simulink model "sampleModel7293_pp_1_1"  (R2018a)
settings: Solver=VariableStepAuto  StartTime=0.0  StopTime=10.0  RelTol=1e-3
undefined symbols (not defined in the file): DiscIntNeverNeededParam
libraries: simulink x367
(part 4 of 12)

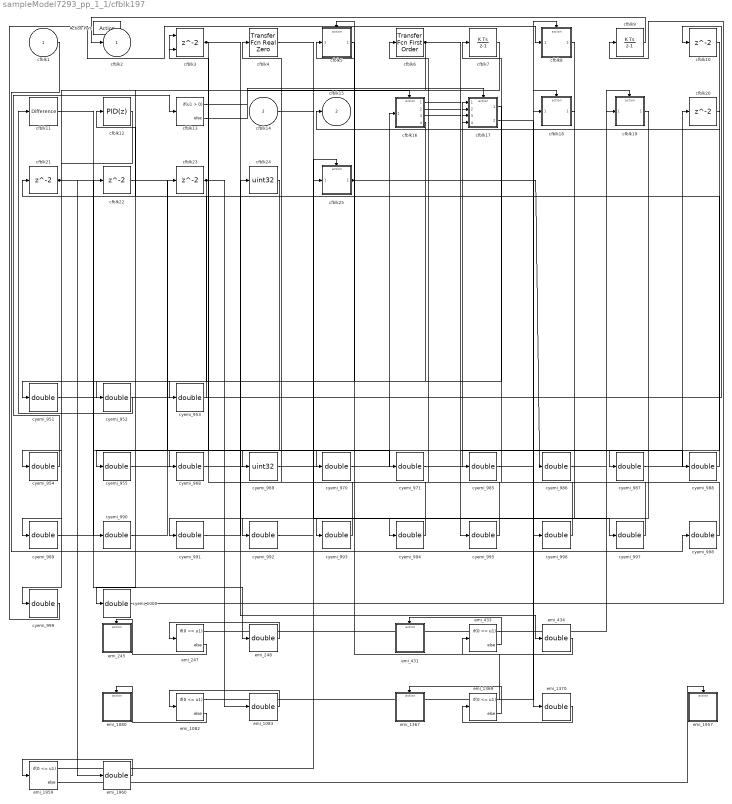
== system sampleModel7293_pp_1_1/cfblk197 ==
  cfblk1 : Inport
  cfblk14 : Inport  Port=2
  Action Port : ActionPort  ActionType=else
  cfblk{10,20..23} (5 alike) : Delay
  cfblk11 : simulink/Discrete/Difference  ICPrevInput=0.0  OutMin=[]  OutMax=[]  OutDataTypeStr=double  OutputDataTypeScalingMode=double  OutDataType=fixdt(1, 16)  OutScaling=2^-10  DoSatur=off
  cfblk12 : simulink/Continuous/PID Controller  Controller=PID  TimeDomain=Discrete-time  SampleTime=-1  IntegratorMethod=Forward Euler  FilterMethod=Forward Euler  Form=Parallel  UseFilter=on  ControllerParametersSource=internal  P=1  I=1  D=0  N=100  InitialConditionSource=internal  InitialConditionForIntegrator=0  InitialConditionForFilter=0  ExternalReset=none  LimitOutput=off  UpperSaturationLimit=inf  LowerSaturationLimit=-inf  LinearizeAsGain=off  AntiWindupMode=none  Kb=1  TrackingMode=off  Kt=1  PParamMin=[]  PParamMax=[]  IParamMin=[]  IParamMax=[]  DParamMin=[]  DParamMax=[]  NParamMin=[]  NParamMax=[]  KbParamMin=[]  KbParamMax=[]  KtParamMin=[]  KtParamMax=[]  POutMin=[]  POutMax=[]  IOutMin=[]  IOutMax=[]  DOutMin=[]  DOutMax=[]  NOutMin=[]  NOutMax=[]  KbOutMin=[]  KbOutMax=[]  KtOutMin=[]  KtOutMax=[]  IntegratorOutMin=[]  IntegratorOutMax=[]  FilterOutMin=[]  FilterOutMax=[]  SumOutMin=[]  SumOutMax=[]  SumI1OutMin=[]  SumI1OutMax=[]  SumI2OutMin=[]  SumI2OutMax=[]  SumI3OutMin=[]  SumI3OutMax=[]  SumDOutMin=[]  SumDOutMax=[]  SaturationOutMin=[]  SaturationOutMax=[]  IntegratorContinuousStateAttributes=''  IntegratorStateMustResolveToSignalObject=off  IntegratorRTWStateStorageClass=Auto  FilterContinuousStateAttributes=''  FilterStateMustResolveToSignalObject=off  FilterRTWStateStorageClass=Auto  DifferentiatorICPrevScaledInput=0  DifferentiatorOutMin=[]  DifferentiatorOutMax=[]  FilterDiffOutCoefMin=[]  FilterDiffOutCoefMax=[]  SumDenOutMin=[]  SumDenOutMax=[]  SumNumOutMin=[]  SumNumOutMax=[]  ReciprocalOutMin=[]  ReciprocalOutMax=[]  DivideOutMin=[]  DivideOutMax=[]  TunerSelectOption=Transfer Function Based (PID Tuner App)
  cfblk13 : If  SampleTime=1
  cfblk16 : Subsystem  TreatAsAtomicUnit=on
  cfblk17 : Subsystem  TreatAsAtomicUnit=on
  cfblk18 : Subsystem  TreatAsAtomicUnit=on
  cfblk19 : Subsystem  TreatAsAtomicUnit=on
  cfblk24 : DataTypeConversion  OutDataTypeStr=uint32
  cfblk25 : Subsystem  TreatAsAtomicUnit=on
  cfblk3 : Delay  ShowEnablePort=on
      settings: InputPortMap=u0,e6
  cfblk4 : simulink/Discrete/Transfer Fcn Real Zero  ZeroZ=0.75  ICPrevInput=0.0  DoSatur=off
      settings: SourceProductName=Simulink  SourceProductBaseCode=SL
  cfblk5 : Subsystem  TreatAsAtomicUnit=on
  cfblk6 : simulink/Discrete/Transfer Fcn First Order  PoleZ=0.95  ICPrevOutput=0.0  DoSatur=off
      settings: SourceProductName=Simulink
  cfblk7 : DiscreteIntegrator  SampleTime=-1  OutDataTypeStr=double  ICPrevOutput=DiscIntNeverNeededParam  ICPrevScaledInput=DiscIntNeverNeededParam
  cfblk8 : Subsystem  TreatAsAtomicUnit=on
  cfblk9 : DiscreteIntegrator  SampleTime=-1  OutDataTypeStr=double  ICPrevOutput=DiscIntNeverNeededParam  ICPrevScaledInput=DiscIntNeverNeededParam
  cyemi_{951..955,968,970..971,985..1000} (24 alike) : DataTypeConversion  OutDataTypeStr=double
  cyemi_969 : DataTypeConversion  OutDataTypeStr=uint32
  emi_1080 : Subsystem  TreatAsAtomicUnit=on
  emi_{247,433,1082,1369,1959} (5 alike) : If  IfExpression=0 <= u1
  emi_{248,434,1083,1370,1960} (5 alike) : DataTypeConversion  OutDataTypeStr=double
  emi_1367 : Subsystem  TreatAsAtomicUnit=on
  emi_1957 : Subsystem  TreatAsAtomicUnit=on
  emi_245 : Subsystem  TreatAsAtomicUnit=on
  emi_431 : Subsystem  TreatAsAtomicUnit=on
  cfblk2 : Outport
  cfblk15 : Outport  Port=2
  wires:
  cfblk10/1 -> cfblk15/1
  cfblk9/1 -> cfblk2/1
  cfblk6/1 -> cyemi_987/1, cyemi_999/1
  cfblk13/1 -> cfblk16/Action
  cfblk13/2 -> cfblk17/Action
  cyemi_951/1 -> cfblk10/1
  cfblk17/1(cfblk2) -> cyemi_951/1
  cyemi_952/1 -> cfblk11/1
  cyemi_953/1 -> cfblk12/1
  cfblk16/4(cfblk13) -> cyemi_953/1
  cyemi_954/1 -> cfblk13/1
  cfblk23/1 -> cyemi_954/1, emi_1083/1
  cyemi_955/1 -> cfblk16/1(cfblk1)
  cfblk20/1 -> cyemi_955/1
  cyemi_968/1 -> cfblk17/1(cfblk1)
  cfblk3/1 -> cyemi_968/1, emi_434/1
  cyemi_969/1 -> cfblk17/2(cfblk12)
  cfblk24/1 -> cyemi_969/1
  cyemi_970/1 -> cfblk17/3(cfblk13)
  cfblk22/1 -> cyemi_970/1
  cyemi_971/1 -> cfblk17/4(cfblk14)
  cfblk21/1 -> cyemi_971/1, emi_248/1, emi_1960/1
  cfblk16/1(cfblk2) -> cyemi_985/1
  cyemi_987/1 -> cfblk20/1
  cyemi_988/1 -> cfblk21/1
  cfblk16/3(cfblk12) -> cyemi_988/1
  cyemi_989/1 -> cfblk22/1
  cfblk12/1 -> cyemi_989/1
  cyemi_990/1 -> cfblk23/1
  cfblk11/1 -> cyemi_990/1
  cyemi_991/1 -> cfblk24/1
  cyemi_993/1 -> cfblk3/1
  cyemi_994/1 -> cfblk3/2
  cfblk14/1 -> cyemi_994/1
  cyemi_995/1 -> cfblk4/1
  cfblk16/2(cfblk11) -> cyemi_995/1
  cfblk17/2(cfblk15) -> cyemi_996/1
  cyemi_997/1 -> cfblk6/1
  cfblk4/1 -> cyemi_997/1
  cyemi_998/1 -> cfblk7/1
  cfblk1/1 -> cyemi_998/1
  cyemi_1000/1 -> cfblk9/1
  cfblk7/1 -> cyemi_1000/1
  cyemi_999/1 -> cfblk8/1(emi_243)
  cfblk8/1(emi_244) -> cyemi_992/1
  emi_247/1 -> cfblk8/Action
  emi_247/2 -> emi_245/Action
  emi_248/1 -> emi_247/1
  cyemi_986/1 -> cfblk19/1(emi_429)
  cfblk19/1(emi_430) -> cyemi_991/1
  emi_433/1 -> cfblk19/Action
  emi_433/2 -> emi_431/Action
  emi_434/1 -> emi_433/1
  cyemi_985/1 -> cfblk18/1(emi_1078)
  cfblk18/1(emi_1079) -> cyemi_993/1
  emi_1082/1 -> cfblk18/Action
  emi_1082/2 -> emi_1080/Action
  emi_1083/1 -> emi_1082/1
  cyemi_996/1 -> cfblk5/1(emi_1365)
  cfblk5/1(emi_1366) -> cyemi_952/1
  emi_1369/1 -> cfblk5/Action
  emi_1369/2 -> emi_1367/Action
  emi_1370/1 -> emi_1369/1
  cyemi_992/1 -> cfblk25/1(emi_1955)
  cfblk25/1(emi_1956) -> emi_1370/1, cyemi_986/1
  emi_1959/1 -> cfblk25/Action
  emi_1959/2 -> emi_1957/Action
  emi_1960/1 -> emi_1959/1

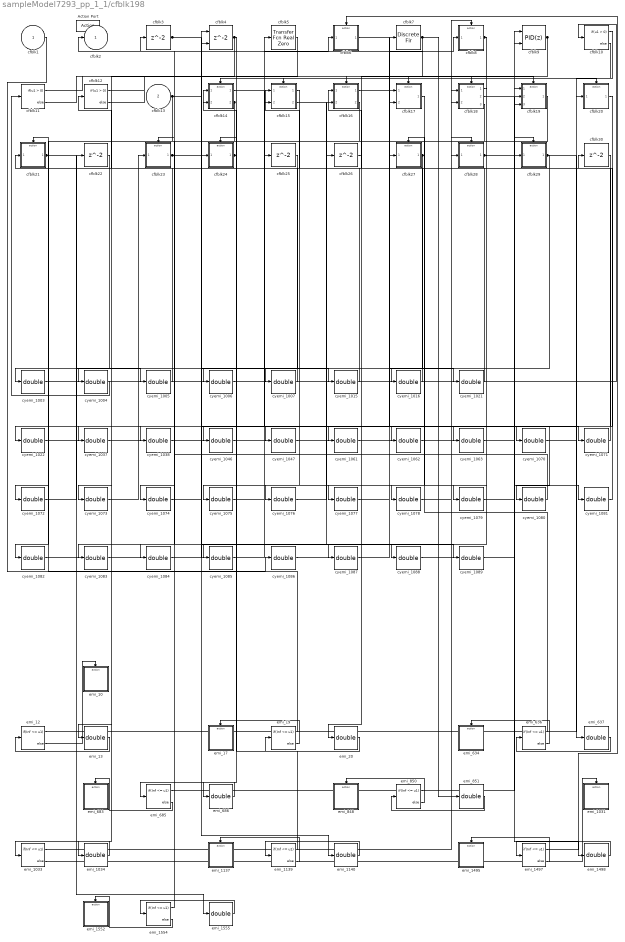
== system sampleModel7293_pp_1_1/cfblk198 ==
  cfblk1 : Inport
  cfblk13 : Inport  Port=2
  Action Port : ActionPort  ActionType=then
  cfblk10 : If  SampleTime=1
  cfblk11 : If  SampleTime=1
  cfblk12 : If  SampleTime=1
  cfblk14 : Subsystem  TreatAsAtomicUnit=on
  cfblk15 : Subsystem  TreatAsAtomicUnit=on
  cfblk16 : Subsystem  TreatAsAtomicUnit=on
  cfblk17 : Subsystem  TreatAsAtomicUnit=on
  cfblk18 : Subsystem  TreatAsAtomicUnit=on
  cfblk19 : Subsystem  TreatAsAtomicUnit=on
  cfblk20 : Subsystem  TreatAsAtomicUnit=on
  cfblk21 : Subsystem  TreatAsAtomicUnit=on
  cfblk{3,22,25..26,30} (5 alike) : Delay
  cfblk23 : Subsystem  TreatAsAtomicUnit=on
  cfblk24 : Subsystem  TreatAsAtomicUnit=on
  cfblk27 : Subsystem  TreatAsAtomicUnit=on
  cfblk28 : Subsystem  TreatAsAtomicUnit=on
  cfblk29 : Subsystem  TreatAsAtomicUnit=on
  cfblk4 : Delay  ShowEnablePort=on
      settings: InputPortMap=u0,e6
  cfblk5 : simulink/Discrete/Transfer Fcn Real Zero  ZeroZ=0.75  ICPrevInput=0.0  DoSatur=off
      settings: SourceProductName=Simulink  SourceProductBaseCode=SL
  cfblk6 : Subsystem  TreatAsAtomicUnit=on
  cfblk7 : DiscreteFir
  cfblk8 : Subsystem  TreatAsAtomicUnit=on
  cfblk9 : simulink/Continuous/PID Controller (2DOF)  Controller=PID  TimeDomain=Discrete-time  SampleTime=-1  IntegratorMethod=Forward Euler  FilterMethod=Forward Euler  Form=Parallel  UseFilter=on  ControllerParametersSource=internal  P=1  I=1  D=0  N=100  b=1  c=1  InitialConditionSource=internal  InitialConditionForIntegrator=0  InitialConditionForFilter=0  ExternalReset=none  LimitOutput=off  UpperSaturationLimit=inf  LowerSaturationLimit=-inf  LinearizeAsGain=off  AntiWindupMode=none  Kb=1  TrackingMode=off  Kt=1  PParamMin=[]  PParamMax=[]  IParamMin=[]  IParamMax=[]  DParamMin=[]  DParamMax=[]  NParamMin=[]  NParamMax=[]  bParamMin=[]  bParamMax=[]  cParamMin=[]  cParamMax=[]  KbParamMin=[]  KbParamMax=[]  KtParamMin=[]  KtParamMax=[]  POutMin=[]  POutMax=[]  IOutMin=[]  IOutMax=[]  DOutMin=[]  DOutMax=[]  NOutMin=[]  NOutMax=[]  bOutMin=[]  bOutMax=[]  cOutMin=[]  cOutMax=[]  KbOutMin=[]  KbOutMax=[]  KtOutMin=[]  KtOutMax=[]  IntegratorOutMin=[]  IntegratorOutMax=[]  FilterOutMin=[]  FilterOutMax=[]  SumOutMin=[]  SumOutMax=[]  Sum1OutMin=[]  Sum1OutMax=[]  Sum2OutMin=[]  Sum2OutMax=[]  Sum3OutMin=[]  Sum3OutMax=[]  SumI1OutMin=[]  SumI1OutMax=[]  SumI2OutMin=[]  SumI2OutMax=[]  SumI3OutMin=[]  SumI3OutMax=[]  SumDOutMin=[]  SumDOutMax=[]  SaturationOutMin=[]  SaturationOutMax=[]  IntegratorContinuousStateAttributes=''  IntegratorStateMustResolveToSignalObject=off  IntegratorRTWStateStorageClass=Auto  FilterContinuousStateAttributes=''  FilterStateMustResolveToSignalObject=off  FilterRTWStateStorageClass=Auto  DifferentiatorICPrevScaledInput=0  DifferentiatorOutMin=[]  DifferentiatorOutMax=[]  FilterDiffOutCoefMin=[]  FilterDiffOutCoefMax=[]  SumDenOutMin=[]  SumDenOutMax=[]  SumNumOutMin=[]  SumNumOutMax=[]  ReciprocalOutMin=[]  ReciprocalOutMax=[]  DivideOutMin=[]  DivideOutMax=[]  TunerSelectOption=Transfer Function Based (PID Tuner App)
  cyemi_{1003..1007,1015..1016,1021..1022,1037..1038,1046..1047,1061..1063,1070..1089} (36 alike) : DataTypeConversion  OutDataTypeStr=double
  emi_10 : Subsystem  TreatAsAtomicUnit=on
  emi_1031 : Subsystem  TreatAsAtomicUnit=on
  emi_{12,19,636,685,850,1033,1139,1497,1554} (9 alike) : If  IfExpression=Inf <= u1
  emi_{13,20,637,686,851,1034,1140,1498,1555} (9 alike) : DataTypeConversion  OutDataTypeStr=double
  emi_1137 : Subsystem  TreatAsAtomicUnit=on
  emi_1495 : Subsystem  TreatAsAtomicUnit=on
  emi_1552 : Subsystem  TreatAsAtomicUnit=on
  emi_17 : Subsystem  TreatAsAtomicUnit=on
  emi_634 : Subsystem  TreatAsAtomicUnit=on
  emi_683 : Subsystem  TreatAsAtomicUnit=on
  emi_848 : Subsystem  TreatAsAtomicUnit=on
  cfblk2 : Outport
  wires:
  cfblk7/1 -> cfblk2/1, emi_20/1, emi_851/1
  cfblk3/1 -> cyemi_1047/1, cyemi_1063/1
  cfblk9/1 -> cyemi_1079/1, cyemi_1087/1
  cfblk13/1 -> cyemi_1004/1, cyemi_1015/1, cyemi_1089/1
  cfblk14/2(cfblk11) -> cyemi_1073/1, cyemi_1074/1
  cfblk10/1 -> cfblk14/Action
  cfblk10/2 -> cfblk15/Action
  cfblk11/1 -> cfblk16/Action
  cfblk11/2 -> cfblk17/Action
  cfblk12/1 -> cfblk18/Action
  cfblk12/2 -> cfblk19/Action
  cyemi_1003/1 -> cfblk10/1
  cyemi_1004/1 -> cfblk11/1
  cyemi_1005/1 -> cfblk12/1
  cyemi_1006/1 -> cfblk14/1(cfblk1)
  cfblk5/1 -> cyemi_1006/1
  cyemi_1007/1 -> cfblk14/2(cfblk10)
  cfblk25/1 -> cyemi_1007/1
  cyemi_1015/1 -> cfblk15/1(cfblk1)
  cyemi_1016/1 -> cfblk15/2(cfblk6)
  cyemi_1021/1 -> cfblk16/1(cfblk1)
  cyemi_1022/1 -> cfblk16/2(cfblk14)
  cyemi_1037/1 -> cfblk17/1(cfblk1)
  cfblk18/3(cfblk16) -> cyemi_1037/1
  cyemi_1038/1 -> cfblk17/2(cfblk10)
  cyemi_1046/1 -> cfblk18/1(cfblk1)
  cyemi_1047/1 -> cfblk18/2(cfblk14)
  cyemi_1061/1 -> cfblk19/1(cfblk1)
  cfblk26/1 -> cyemi_1061/1
  cyemi_1062/1 -> cfblk19/2(cfblk9)
  cyemi_1063/1 -> cfblk19/3(cfblk10)
  cfblk16/1(cfblk2) -> cyemi_1070/1
  cfblk14/1(cfblk2) -> cyemi_1071/1
  cyemi_1072/1 -> cfblk22/1
  cfblk19/1(cfblk2) -> cyemi_1072/1
  cyemi_1075/1 -> cfblk25/1
  cfblk15/1(cfblk2) -> cyemi_1075/1
  cyemi_1076/1 -> cfblk26/1
  cfblk17/1(cfblk2) -> cyemi_1078/1
  cyemi_1080/1 -> cfblk3/1
  cfblk30/1 -> cyemi_1080/1
  cyemi_1081/1 -> cfblk30/1
  cfblk18/2(cfblk15) -> cyemi_1081/1
  cyemi_1082/1 -> cfblk4/1
  cfblk22/1 -> cyemi_1082/1
  cyemi_1083/1 -> cfblk4/2
  cfblk18/1(cfblk2) -> cyemi_1083/1
  cyemi_1084/1 -> cfblk5/1
  cfblk16/2(cfblk15) -> cyemi_1084/1
  cfblk4/1 -> cyemi_1085/1, emi_13/1
  cyemi_1086/1 -> cfblk7/1
  cfblk1/1 -> cyemi_1086/1
  cyemi_1088/1 -> cfblk9/1
  cfblk15/2(cfblk7) -> cyemi_1088/1
  cyemi_1089/1 -> cfblk9/2
  cyemi_1070/1 -> cfblk20/1(emi_8)
  cfblk20/1(emi_9) -> cyemi_1046/1
  emi_12/1 -> cfblk20/Action
  emi_12/2 -> emi_10/Action
  emi_13/1 -> emi_12/1
  cyemi_1071/1 -> cfblk21/1(emi_15)
  cfblk21/1(emi_16) -> cyemi_1005/1, emi_1555/1
  emi_19/1 -> cfblk21/Action
  emi_19/2 -> emi_17/Action
  emi_20/1 -> emi_19/1
  cyemi_1077/1 -> cfblk27/1(emi_632)
  cfblk27/1(emi_633) -> cyemi_1038/1, emi_1034/1
  emi_636/1 -> cfblk27/Action
  emi_636/2 -> emi_634/Action
  emi_637/1 -> emi_636/1
  cyemi_1079/1 -> cfblk29/1(emi_681)
  cfblk29/1(emi_682) -> emi_637/1, cyemi_1016/1
  emi_685/1 -> cfblk29/Action
  emi_685/2 -> emi_683/Action
  emi_686/1 -> emi_685/1
  cyemi_1087/1 -> cfblk8/1(emi_846)
  cfblk8/1(emi_847) -> cyemi_1077/1, cyemi_1076/1
  emi_850/1 -> cfblk8/Action
  emi_850/2 -> emi_848/Action
  emi_851/1 -> emi_850/1
  cyemi_1078/1 -> cfblk28/1(emi_1029)
  cfblk28/1(emi_1030) -> cyemi_1062/1, emi_1498/1
  emi_1033/1 -> cfblk28/Action
  emi_1033/2 -> emi_1031/Action
  emi_1034/1 -> emi_1033/1
  cyemi_1074/1 -> cfblk24/1(emi_1135)
  cfblk24/1(emi_1136) -> emi_686/1, cyemi_1003/1
  emi_1139/1 -> cfblk24/Action
  emi_1139/2 -> emi_1137/Action
  emi_1140/1 -> emi_1139/1
  cyemi_1085/1 -> cfblk6/1(emi_1493)
  cfblk6/1(emi_1494) -> cyemi_1021/1
  emi_1497/1 -> cfblk6/Action
  emi_1497/2 -> emi_1495/Action
  emi_1498/1 -> emi_1497/1
  cyemi_1073/1 -> cfblk23/1(emi_1550)
  cfblk23/1(emi_1551) -> emi_1140/1, cyemi_1022/1
  emi_1554/1 -> cfblk23/Action
  emi_1554/2 -> emi_1552/Action
  emi_1555/1 -> emi_1554/1

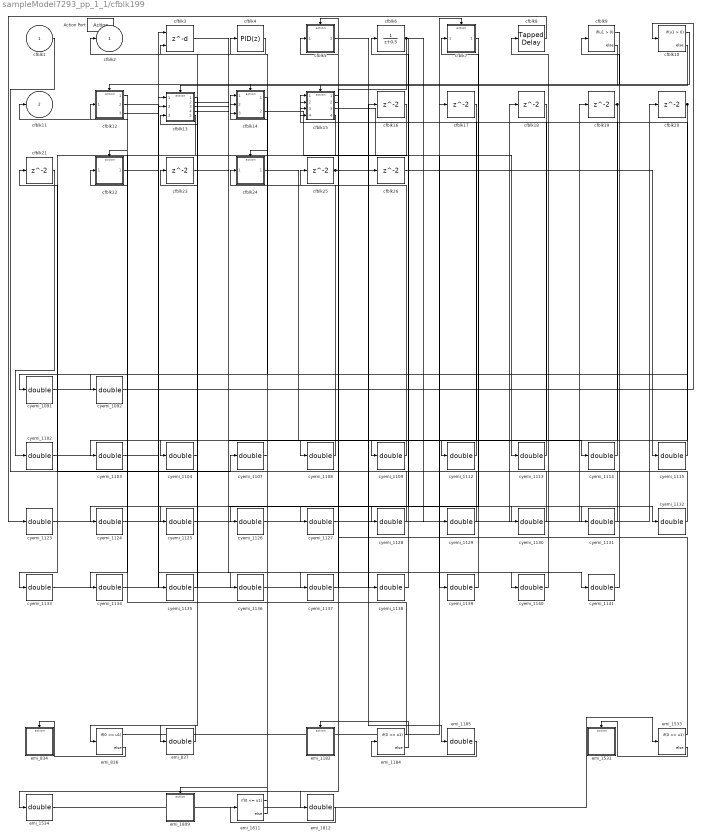
== system sampleModel7293_pp_1_1/cfblk199 ==
  cfblk1 : Inport
  Action Port : ActionPort  ActionType=else
  cfblk10 : If  SampleTime=1
  cfblk12 : Subsystem  TreatAsAtomicUnit=on
  cfblk13 : Subsystem  TreatAsAtomicUnit=on
  cfblk14 : Subsystem  TreatAsAtomicUnit=on
  cfblk15 : Subsystem  TreatAsAtomicUnit=on
  cfblk{16..21,23,25..26} (9 alike) : Delay
  cfblk22 : Subsystem  TreatAsAtomicUnit=on
  cfblk24 : Subsystem  TreatAsAtomicUnit=on
  cfblk3 : Delay  DelayLengthSource=Input port
      settings: InputPortMap=u0,p1
  cfblk4 : simulink/Continuous/PID Controller  Controller=PID  TimeDomain=Discrete-time  SampleTime=-1  IntegratorMethod=Forward Euler  FilterMethod=Forward Euler  Form=Parallel  UseFilter=on  ControllerParametersSource=internal  P=1  I=1  D=0  N=100  InitialConditionSource=internal  InitialConditionForIntegrator=0  InitialConditionForFilter=0  ExternalReset=none  LimitOutput=off  UpperSaturationLimit=inf  LowerSaturationLimit=-inf  LinearizeAsGain=off  AntiWindupMode=none  Kb=1  TrackingMode=off  Kt=1  PParamMin=[]  PParamMax=[]  IParamMin=[]  IParamMax=[]  DParamMin=[]  DParamMax=[]  NParamMin=[]  NParamMax=[]  KbParamMin=[]  KbParamMax=[]  KtParamMin=[]  KtParamMax=[]  POutMin=[]  POutMax=[]  IOutMin=[]  IOutMax=[]  DOutMin=[]  DOutMax=[]  NOutMin=[]  NOutMax=[]  KbOutMin=[]  KbOutMax=[]  KtOutMin=[]  KtOutMax=[]  IntegratorOutMin=[]  IntegratorOutMax=[]  FilterOutMin=[]  FilterOutMax=[]  SumOutMin=[]  SumOutMax=[]  SumI1OutMin=[]  SumI1OutMax=[]  SumI2OutMin=[]  SumI2OutMax=[]  SumI3OutMin=[]  SumI3OutMax=[]  SumDOutMin=[]  SumDOutMax=[]  SaturationOutMin=[]  SaturationOutMax=[]  IntegratorContinuousStateAttributes=''  IntegratorStateMustResolveToSignalObject=off  IntegratorRTWStateStorageClass=Auto  FilterContinuousStateAttributes=''  FilterStateMustResolveToSignalObject=off  FilterRTWStateStorageClass=Auto  DifferentiatorICPrevScaledInput=0  DifferentiatorOutMin=[]  DifferentiatorOutMax=[]  FilterDiffOutCoefMin=[]  FilterDiffOutCoefMax=[]  SumDenOutMin=[]  SumDenOutMax=[]  SumNumOutMin=[]  SumNumOutMax=[]  ReciprocalOutMin=[]  ReciprocalOutMax=[]  DivideOutMin=[]  DivideOutMax=[]  TunerSelectOption=Transfer Function Based (PID Tuner App)
  cfblk5 : Subsystem  TreatAsAtomicUnit=on
  cfblk6 : DiscreteTransferFcn
  cfblk7 : Subsystem  TreatAsAtomicUnit=on
  cfblk8 : simulink/Discrete/Tapped Delay  vinit=0.0  samptime=-1  NumDelays=1  DelayOrder=Oldest  includeCurrent=off
  cfblk9 : If  SampleTime=1
  cyemi_{1091..1092,1102..1104,1107..1109,1112..1115,1123..1141} (31 alike) : DataTypeConversion  OutDataTypeStr=double
  emi_1182 : Subsystem  TreatAsAtomicUnit=on
  emi_{836,1184,1533,1811} (4 alike) : If  IfExpression=0 <= u1
  emi_{837,1185,1534,1812} (4 alike) : DataTypeConversion  OutDataTypeStr=double
  emi_1531 : Subsystem  TreatAsAtomicUnit=on
  emi_1809 : Subsystem  TreatAsAtomicUnit=on
  emi_834 : Subsystem  TreatAsAtomicUnit=on
  cfblk2 : Outport
  cfblk11 : Outport  Port=2
  wires:
  cfblk12/1(cfblk2) -> cfblk11/1
  cfblk6/1 -> cyemi_1128/1, cyemi_1129/1, emi_1534/1
  cfblk4/1 -> cfblk2/1
  cfblk9/1 -> cfblk12/Action
  cfblk9/2 -> cfblk13/Action
  cfblk10/1 -> cfblk14/Action
  cfblk10/2 -> cfblk15/Action
  cyemi_1091/1 -> cfblk10/1
  cfblk20/1 -> cyemi_1091/1, emi_837/1
  cyemi_1092/1 -> cfblk12/1(cfblk1)
  cfblk14/1(cfblk2) -> cyemi_1092/1
  cyemi_1102/1 -> cfblk13/1(cfblk1)
  cfblk21/1 -> cyemi_1102/1
  cyemi_1103/1 -> cfblk13/2(cfblk5)
  cfblk18/1 -> cyemi_1103/1
  cyemi_1104/1 -> cfblk13/3(cfblk6)
  cfblk16/1 -> cyemi_1104/1
  cyemi_1107/1 -> cfblk14/1(cfblk1)
  cfblk1/1 -> cyemi_1107/1
  cyemi_1108/1 -> cfblk14/2(cfblk5)
  cfblk23/1 -> cyemi_1108/1
  cyemi_1109/1 -> cfblk14/3(cfblk6)
  cfblk19/1 -> cyemi_1109/1, emi_1812/1
  cyemi_1112/1 -> cfblk15/1(cfblk1)
  cfblk17/1 -> cyemi_1112/1
  cyemi_1113/1 -> cfblk15/2(cfblk9)
  cfblk14/2(cfblk7) -> cyemi_1113/1
  cyemi_1114/1 -> cfblk15/3(cfblk10)
  cyemi_1115/1 -> cfblk15/4(cfblk11)
  cfblk26/1 -> cyemi_1115/1
  cyemi_1123/1 -> cfblk16/1
  cfblk8/1 -> cyemi_1123/1
  cyemi_1124/1 -> cfblk17/1
  cfblk13/1(cfblk2) -> cyemi_1124/1
  cyemi_1125/1 -> cfblk18/1
  cfblk15/1(cfblk2) -> cyemi_1125/1
  cyemi_1126/1 -> cfblk19/1
  cfblk15/2(cfblk12) -> cyemi_1126/1
  cyemi_1127/1 -> cfblk20/1
  cyemi_1128/1 -> cfblk21/1
  cyemi_1130/1 -> cfblk23/1
  cfblk13/2(cfblk7) -> cyemi_1130/1
  cfblk13/3(cfblk8) -> cyemi_1131/1
  cyemi_1132/1 -> cfblk25/1
  cfblk13/4(cfblk9) -> cyemi_1132/1
  cyemi_1133/1 -> cfblk26/1
  cfblk13/5(cfblk10) -> cyemi_1133/1
  cyemi_1134/1 -> cfblk3/1
  cfblk15/4(cfblk14) -> cyemi_1134/1
  cyemi_1135/1 -> cfblk3/2
  cyemi_1136/1 -> cfblk4/1
  cfblk12/2(cfblk9) -> cyemi_1136/1
  cfblk3/1 -> cyemi_1137/1
  cyemi_1138/1 -> cfblk6/1
  cfblk15/3(cfblk13) -> cyemi_1139/1
  cyemi_1140/1 -> cfblk8/1
  cfblk12/3(cfblk10) -> cyemi_1140/1
  cyemi_1141/1 -> cfblk9/1
  cfblk25/1 -> cyemi_1141/1, emi_1185/1
  cyemi_1139/1 -> cfblk7/1(emi_832)
  cfblk7/1(emi_833) -> cyemi_1127/1
  emi_836/1 -> cfblk7/Action
  emi_836/2 -> emi_834/Action
  emi_837/1 -> emi_836/1
  cyemi_1129/1 -> cfblk22/1(emi_1180)
  cfblk22/1(emi_1181) -> cyemi_1135/1
  emi_1184/1 -> cfblk22/Action
  emi_1184/2 -> emi_1182/Action
  emi_1185/1 -> emi_1184/1
  cyemi_1137/1 -> cfblk5/1(emi_1529)
  cfblk5/1(emi_1530) -> cyemi_1138/1
  emi_1533/1 -> cfblk5/Action
  emi_1533/2 -> emi_1531/Action
  emi_1534/1 -> emi_1533/1
  cyemi_1131/1 -> cfblk24/1(emi_1807)
  cfblk24/1(emi_1808) -> cyemi_1114/1
  emi_1811/1 -> cfblk24/Action
  emi_1811/2 -> emi_1809/Action
  emi_1812/1 -> emi_1811/1

== system sampleModel7293_pp_1_1/cfblk2 ==
  emi_1245 : Inport
  Action Port : ActionPort  ActionType=then
  cfblk2 : DiscreteIntegrator  OutDataTypeStr=double  ICPrevOutput=DiscIntNeverNeededParam  ICPrevScaledInput=DiscIntNeverNeededParam
  emi_1246 : Outport
  wires:
  emi_1245/1 -> cfblk2/1
  cfblk2/1 -> emi_1246/1

== system sampleModel7293_pp_1_1/cfblk200 ==
  cfblk1 : Inport
  Action Port : ActionPort  ActionType=then
  cfblk10 : If  SampleTime=1
  cfblk11 : Subsystem  TreatAsAtomicUnit=on
  cfblk12 : Subsystem  TreatAsAtomicUnit=on
  cfblk13 : Delay
  cfblk14 : Delay
  cfblk3 : Subsystem  TreatAsAtomicUnit=on
  cfblk4 : Subsystem  TreatAsAtomicUnit=on
  cfblk5 : Delay  DelayLengthSource=Input port
      settings: InputPortMap=u0,p1
  cfblk6 : Delay
  cfblk7 : UnitDelay  SampleTime=-1
  cfblk8 : simulink/Continuous/PID Controller (2DOF)  Controller=PID  TimeDomain=Discrete-time  SampleTime=-1  IntegratorMethod=Forward Euler  FilterMethod=Forward Euler  Form=Parallel  UseFilter=on  ControllerParametersSource=internal  P=1  I=1  D=0  N=100  b=1  c=1  InitialConditionSource=internal  InitialConditionForIntegrator=0  InitialConditionForFilter=0  ExternalReset=none  LimitOutput=off  UpperSaturationLimit=inf  LowerSaturationLimit=-inf  LinearizeAsGain=off  AntiWindupMode=none  Kb=1  TrackingMode=off  Kt=1  PParamMin=[]  PParamMax=[]  IParamMin=[]  IParamMax=[]  DParamMin=[]  DParamMax=[]  NParamMin=[]  NParamMax=[]  bParamMin=[]  bParamMax=[]  cParamMin=[]  cParamMax=[]  KbParamMin=[]  KbParamMax=[]  KtParamMin=[]  KtParamMax=[]  POutMin=[]  POutMax=[]  IOutMin=[]  IOutMax=[]  DOutMin=[]  DOutMax=[]  NOutMin=[]  NOutMax=[]  bOutMin=[]  bOutMax=[]  cOutMin=[]  cOutMax=[]  KbOutMin=[]  KbOutMax=[]  KtOutMin=[]  KtOutMax=[]  IntegratorOutMin=[]  IntegratorOutMax=[]  FilterOutMin=[]  FilterOutMax=[]  SumOutMin=[]  SumOutMax=[]  Sum1OutMin=[]  Sum1OutMax=[]  Sum2OutMin=[]  Sum2OutMax=[]  Sum3OutMin=[]  Sum3OutMax=[]  SumI1OutMin=[]  SumI1OutMax=[]  SumI2OutMin=[]  SumI2OutMax=[]  SumI3OutMin=[]  SumI3OutMax=[]  SumDOutMin=[]  SumDOutMax=[]  SaturationOutMin=[]  SaturationOutMax=[]  IntegratorContinuousStateAttributes=''  IntegratorStateMustResolveToSignalObject=off  IntegratorRTWStateStorageClass=Auto  FilterContinuousStateAttributes=''  FilterStateMustResolveToSignalObject=off  FilterRTWStateStorageClass=Auto  DifferentiatorICPrevScaledInput=0  DifferentiatorOutMin=[]  DifferentiatorOutMax=[]  FilterDiffOutCoefMin=[]  FilterDiffOutCoefMax=[]  SumDenOutMin=[]  SumDenOutMax=[]  SumNumOutMin=[]  SumNumOutMax=[]  ReciprocalOutMin=[]  ReciprocalOutMax=[]  DivideOutMin=[]  DivideOutMax=[]  TunerSelectOption=Transfer Function Based (PID Tuner App)
  cfblk9 : UnitDelay  SampleTime=-1
  cyemi_{1145..1146,1157..1158,1169..1179} (15 alike) : DataTypeConversion  OutDataTypeStr=double
  emi_641 : Subsystem  TreatAsAtomicUnit=on
  emi_643 : If  IfExpression=Inf <= u1
  emi_644 : DataTypeConversion  OutDataTypeStr=double
  emi_926 : Subsystem  TreatAsAtomicUnit=on
  emi_928 : If  IfExpression=Inf <= u1
  emi_929 : DataTypeConversion  OutDataTypeStr=double
  cfblk2 : Outport
  wires:
  cfblk9/1 -> cfblk2/1, emi_929/1
  cfblk5/1 -> cyemi_1158/1, cyemi_1176/1
  cfblk6/1 -> cyemi_1174/1, cyemi_1179/1, emi_644/1
  cfblk10/1 -> cfblk11/Action
  cfblk10/2 -> cfblk12/Action
  cyemi_1145/1 -> cfblk10/1
  cyemi_1146/1 -> cfblk11/1(cfblk1)
  cfblk14/1 -> cyemi_1146/1
  cyemi_1157/1 -> cfblk12/1(cfblk1)
  cyemi_1158/1 -> cfblk12/2(cfblk9)
  cyemi_1169/1 -> cfblk13/1
  cfblk8/1 -> cyemi_1169/1
  cyemi_1170/1 -> cfblk14/1
  cfblk7/1 -> cyemi_1171/1
  cfblk11/1(cfblk2) -> cyemi_1172/1
  cyemi_1173/1 -> cfblk5/1
  cfblk13/1 -> cyemi_1173/1
  cyemi_1174/1 -> cfblk5/2
  cyemi_1175/1 -> cfblk6/1
  cfblk1/1 -> cyemi_1175/1
  cyemi_1176/1 -> cfblk7/1
  cyemi_1177/1 -> cfblk8/1
  cfblk12/1(cfblk2) -> cyemi_1177/1
  cyemi_1178/1 -> cfblk8/2
  cyemi_1179/1 -> cfblk9/1
  cyemi_1172/1 -> cfblk4/1(emi_639)
  cfblk4/1(emi_640) -> cyemi_1170/1
  emi_643/1 -> cfblk4/Action
  emi_643/2 -> emi_641/Action
  emi_644/1 -> emi_643/1
  cyemi_1171/1 -> cfblk3/1(emi_924)
  cfblk3/1(emi_925) -> cyemi_1178/1, cyemi_1157/1, cyemi_1145/1
  emi_928/1 -> cfblk3/Action
  emi_928/2 -> emi_926/Action
  emi_929/1 -> emi_928/1

== system sampleModel7293_pp_1_1/cfblk201 ==
  cfblk1 : Inport
  Action Port : ActionPort  ActionType=else
  cfblk10 : simulink/Discrete/Transfer Fcn First Order  PoleZ=0.95  ICPrevOutput=0.0  DoSatur=off
      settings: SourceProductName=Simulink
  cfblk11 : DiscreteIntegrator  SampleTime=-1  OutDataTypeStr=double  ICPrevOutput=DiscIntNeverNeededParam  ICPrevScaledInput=DiscIntNeverNeededParam
  cfblk12 : Subsystem  TreatAsAtomicUnit=on
  cfblk13 : simulink/Discrete/Transfer Fcn Real Zero  ZeroZ=0.75  ICPrevInput=0.0  DoSatur=off
      settings: SourceProductName=Simulink  SourceProductBaseCode=SL
  cfblk14 : DiscreteStateSpace  SampleTime=-1
  cfblk15 : Delay
  cfblk3 : UnitDelay  SampleTime=-1
  cfblk4 : Subsystem  TreatAsAtomicUnit=on
  cfblk5 : DiscreteFir
  cfblk6 : DiscreteTransferFcn
  cfblk7 : Subsystem  TreatAsAtomicUnit=on
  cfblk8 : Subsystem  TreatAsAtomicUnit=on
  cfblk9 : Delay
  cyemi_{1181..1194} (14 alike) : DataTypeConversion  OutDataTypeStr=double
  emi_1261 : Subsystem  TreatAsAtomicUnit=on
  emi_{477,914,1263,1312} (4 alike) : If  IfExpression=0 <= u1
  emi_{478,915,1264,1313} (4 alike) : DataTypeConversion  OutDataTypeStr=double
  emi_1310 : Subsystem  TreatAsAtomicUnit=on
  emi_475 : Subsystem  TreatAsAtomicUnit=on
  emi_912 : Subsystem  TreatAsAtomicUnit=on
  cfblk2 : Outport
  wires:
  cfblk1/1 -> cyemi_1189/1, cyemi_1190/1
  cfblk13/1 -> cfblk2/1
  cyemi_1181/1 -> cfblk10/1
  cfblk14/1 -> cyemi_1181/1
  cyemi_1182/1 -> cfblk11/1
  cfblk6/1 -> cyemi_1183/1
  cyemi_1184/1 -> cfblk13/1
  cyemi_1185/1 -> cfblk14/1
  cyemi_1186/1 -> cfblk15/1
  cfblk9/1 -> cyemi_1186/1, emi_1313/1
  cyemi_1187/1 -> cfblk3/1
  cfblk11/1 -> cyemi_1187/1
  cfblk3/1 -> cyemi_1188/1
  cyemi_1190/1 -> cfblk5/1
  cyemi_1191/1 -> cfblk6/1
  cfblk5/1 -> cyemi_1192/1, emi_915/1
  cfblk15/1 -> cyemi_1193/1, emi_1264/1
  cyemi_1194/1 -> cfblk9/1
  cfblk10/1 -> cyemi_1194/1
  cyemi_1188/1 -> cfblk4/1(emi_472)
  cyemi_1189/1 -> cfblk4/2(emi_473)
  cfblk4/1(emi_474) -> cyemi_1184/1
  emi_477/1 -> cfblk4/Action
  emi_477/2 -> emi_475/Action
  emi_478/1 -> emi_477/1
  cyemi_1192/1 -> cfblk7/1(emi_910)
  cfblk7/1(emi_911) -> cyemi_1191/1
  emi_914/1 -> cfblk7/Action
  emi_914/2 -> emi_912/Action
  emi_915/1 -> emi_914/1
  cyemi_1183/1 -> cfblk12/1(emi_1259)
  cfblk12/1(emi_1260) -> cyemi_1182/1
  emi_1263/1 -> cfblk12/Action
  emi_1263/2 -> emi_1261/Action
  emi_1264/1 -> emi_1263/1
  cyemi_1193/1 -> cfblk8/1(emi_1308)
  cfblk8/1(emi_1309) -> emi_478/1, cyemi_1185/1
  emi_1312/1 -> cfblk8/Action
  emi_1312/2 -> emi_1310/Action
  emi_1313/1 -> emi_1312/1

== system sampleModel7293_pp_1_1/cfblk202 ==
  cfblk1 : Inport
  Action Port : ActionPort  ActionType=then
  cfblk10 : Subsystem  TreatAsAtomicUnit=on
  cfblk11 : DiscreteTransferFcn
  cfblk12 : Delay
  cfblk13 : Subsystem  TreatAsAtomicUnit=on
  cfblk3 : Subsystem  TreatAsAtomicUnit=on
  cfblk4 : Subsystem  TreatAsAtomicUnit=on
  cfblk5 : simulink/Continuous/PID Controller (2DOF)  Controller=PID  TimeDomain=Discrete-time  SampleTime=-1  IntegratorMethod=Forward Euler  FilterMethod=Forward Euler  Form=Parallel  UseFilter=on  ControllerParametersSource=internal  P=1  I=1  D=0  N=100  b=1  c=1  InitialConditionSource=internal  InitialConditionForIntegrator=0  InitialConditionForFilter=0  ExternalReset=none  LimitOutput=off  UpperSaturationLimit=inf  LowerSaturationLimit=-inf  LinearizeAsGain=off  AntiWindupMode=none  Kb=1  TrackingMode=off  Kt=1  PParamMin=[]  PParamMax=[]  IParamMin=[]  IParamMax=[]  DParamMin=[]  DParamMax=[]  NParamMin=[]  NParamMax=[]  bParamMin=[]  bParamMax=[]  cParamMin=[]  cParamMax=[]  KbParamMin=[]  KbParamMax=[]  KtParamMin=[]  KtParamMax=[]  POutMin=[]  POutMax=[]  IOutMin=[]  IOutMax=[]  DOutMin=[]  DOutMax=[]  NOutMin=[]  NOutMax=[]  bOutMin=[]  bOutMax=[]  cOutMin=[]  cOutMax=[]  KbOutMin=[]  KbOutMax=[]  KtOutMin=[]  KtOutMax=[]  IntegratorOutMin=[]  IntegratorOutMax=[]  FilterOutMin=[]  FilterOutMax=[]  SumOutMin=[]  SumOutMax=[]  Sum1OutMin=[]  Sum1OutMax=[]  Sum2OutMin=[]  Sum2OutMax=[]  Sum3OutMin=[]  Sum3OutMax=[]  SumI1OutMin=[]  SumI1OutMax=[]  SumI2OutMin=[]  SumI2OutMax=[]  SumI3OutMin=[]  SumI3OutMax=[]  SumDOutMin=[]  SumDOutMax=[]  SaturationOutMin=[]  SaturationOutMax=[]  IntegratorContinuousStateAttributes=''  IntegratorStateMustResolveToSignalObject=off  IntegratorRTWStateStorageClass=Auto  FilterContinuousStateAttributes=''  FilterStateMustResolveToSignalObject=off  FilterRTWStateStorageClass=Auto  DifferentiatorICPrevScaledInput=0  DifferentiatorOutMin=[]  DifferentiatorOutMax=[]  FilterDiffOutCoefMin=[]  FilterDiffOutCoefMax=[]  SumDenOutMin=[]  SumDenOutMax=[]  SumNumOutMin=[]  SumNumOutMax=[]  ReciprocalOutMin=[]  ReciprocalOutMax=[]  DivideOutMin=[]  DivideOutMax=[]  TunerSelectOption=Transfer Function Based (PID Tuner App)
  cfblk6 : UnitDelay  SampleTime=-1
  cfblk7 : Subsystem  TreatAsAtomicUnit=on
  cfblk8 : Delay  DelayLengthSource=Input port
      settings: InputPortMap=u0,p1
  cfblk9 : simulink/Continuous/PID Controller (2DOF)  Controller=PID  TimeDomain=Discrete-time  SampleTime=-1  IntegratorMethod=Forward Euler  FilterMethod=Forward Euler  Form=Parallel  UseFilter=on  ControllerParametersSource=internal  P=1  I=1  D=0  N=100  b=1  c=1  InitialConditionSource=internal  InitialConditionForIntegrator=0  InitialConditionForFilter=0  ExternalReset=none  LimitOutput=off  UpperSaturationLimit=inf  LowerSaturationLimit=-inf  LinearizeAsGain=off  AntiWindupMode=none  Kb=1  TrackingMode=off  Kt=1  PParamMin=[]  PParamMax=[]  IParamMin=[]  IParamMax=[]  DParamMin=[]  DParamMax=[]  NParamMin=[]  NParamMax=[]  bParamMin=[]  bParamMax=[]  cParamMin=[]  cParamMax=[]  KbParamMin=[]  KbParamMax=[]  KtParamMin=[]  KtParamMax=[]  POutMin=[]  POutMax=[]  IOutMin=[]  IOutMax=[]  DOutMin=[]  DOutMax=[]  NOutMin=[]  NOutMax=[]  bOutMin=[]  bOutMax=[]  cOutMin=[]  cOutMax=[]  KbOutMin=[]  KbOutMax=[]  KtOutMin=[]  KtOutMax=[]  IntegratorOutMin=[]  IntegratorOutMax=[]  FilterOutMin=[]  FilterOutMax=[]  SumOutMin=[]  SumOutMax=[]  Sum1OutMin=[]  Sum1OutMax=[]  Sum2OutMin=[]  Sum2OutMax=[]  Sum3OutMin=[]  Sum3OutMax=[]  SumI1OutMin=[]  SumI1OutMax=[]  SumI2OutMin=[]  SumI2OutMax=[]  SumI3OutMin=[]  SumI3OutMax=[]  SumDOutMin=[]  SumDOutMax=[]  SaturationOutMin=[]  SaturationOutMax=[]  IntegratorContinuousStateAttributes=''  IntegratorStateMustResolveToSignalObject=off  IntegratorRTWStateStorageClass=Auto  FilterContinuousStateAttributes=''  FilterStateMustResolveToSignalObject=off  FilterRTWStateStorageClass=Auto  DifferentiatorICPrevScaledInput=0  DifferentiatorOutMin=[]  DifferentiatorOutMax=[]  FilterDiffOutCoefMin=[]  FilterDiffOutCoefMax=[]  SumDenOutMin=[]  SumDenOutMax=[]  SumNumOutMin=[]  SumNumOutMax=[]  ReciprocalOutMin=[]  ReciprocalOutMax=[]  DivideOutMin=[]  DivideOutMax=[]  TunerSelectOption=Transfer Function Based (PID Tuner App)
  cyemi_{1196..1209} (14 alike) : DataTypeConversion  OutDataTypeStr=double
  emi_1167 : Subsystem  TreatAsAtomicUnit=on
  emi_{585,963,1169,1526,1739} (5 alike) : If  IfExpression=0 <= u1
  emi_{586,964,1170,1527,1740} (5 alike) : DataTypeConversion  OutDataTypeStr=double
  emi_1524 : Subsystem  TreatAsAtomicUnit=on
  emi_1737 : Subsystem  TreatAsAtomicUnit=on
  emi_583 : Subsystem  TreatAsAtomicUnit=on
  emi_961 : Subsystem  TreatAsAtomicUnit=on
  cfblk2 : Outport
  wires:
  cfblk9/1 -> cfblk2/1
  cfblk11/1 -> cyemi_1199/1, cyemi_1202/1
  cfblk1/1 -> cyemi_1196/1
  cyemi_1197/1 -> cfblk11/1
  cfblk6/1 -> cyemi_1197/1
  cyemi_1198/1 -> cfblk12/1
  cfblk12/1 -> cyemi_1200/1
  cyemi_1202/1 -> cfblk5/1
  cyemi_1203/1 -> cfblk5/2
  cyemi_1204/1 -> cfblk6/1
  cyemi_1206/1 -> cfblk8/1
  cfblk5/1 -> cyemi_1206/1
  cyemi_1207/1 -> cfblk8/2
  cyemi_1208/1 -> cfblk9/1
  cfblk8/1 -> cyemi_1208/1, emi_586/1, emi_1170/1, emi_1527/1
  cyemi_1209/1 -> cfblk9/2
  cyemi_1201/1 -> cfblk4/1(emi_581)
  cfblk4/1(emi_582) -> cyemi_1198/1
  emi_585/1 -> cfblk4/Action
  emi_585/2 -> emi_583/Action
  emi_586/1 -> emi_585/1
  cyemi_1200/1 -> cfblk3/1(emi_959)
  cfblk3/1(emi_960) -> cyemi_1209/1, cyemi_1203/1, cyemi_1201/1
  emi_963/1 -> cfblk3/Action
  emi_963/2 -> emi_961/Action
  emi_964/1 -> emi_963/1
  cyemi_1205/1 -> cfblk7/1(emi_1165)
  cfblk7/1(emi_1166) -> emi_964/1, cyemi_1207/1, emi_1740/1
  emi_1169/1 -> cfblk7/Action
  emi_1169/2 -> emi_1167/Action
  emi_1170/1 -> emi_1169/1
  cyemi_1199/1 -> cfblk13/1(emi_1522)
  cfblk13/1(emi_1523) -> cyemi_1204/1
  emi_1526/1 -> cfblk13/Action
  emi_1526/2 -> emi_1524/Action
  emi_1527/1 -> emi_1526/1
  cyemi_1196/1 -> cfblk10/1(emi_1735)
  cfblk10/1(emi_1736) -> cyemi_1205/1
  emi_1739/1 -> cfblk10/Action
  emi_1739/2 -> emi_1737/Action
  emi_1740/1 -> emi_1739/1

== system sampleModel7293_pp_1_1/cfblk203 ==
  cfblk1 : Inport
  Action Port : ActionPort  ActionType=else
  cfblk10 : simulink/Discrete/Transfer Fcn Lead or Lag  PoleZ=0.95  ZeroZ=0.75  ICPrevOutput=0.0  ICPrevInput=0.0  DoSatur=off
      settings: SourceProductName=Simulink  SourceProductBaseCode=SL
  cfblk11 : If  SampleTime=1
  cfblk12 : Subsystem  TreatAsAtomicUnit=on
  cfblk13 : Subsystem  TreatAsAtomicUnit=on
  cfblk14 : Delay
  cfblk15 : Delay
  cfblk16 : Subsystem  TreatAsAtomicUnit=on
  cfblk17 : Subsystem  TreatAsAtomicUnit=on
  cfblk3 : DiscreteIntegrator  SampleTime=-1  OutDataTypeStr=double  ICPrevOutput=DiscIntNeverNeededParam  ICPrevScaledInput=DiscIntNeverNeededParam
  cfblk4 : Delay  ShowEnablePort=on
      settings: InputPortMap=u0,e6
  cfblk5 : simulink/Continuous/PID Controller  Controller=PID  TimeDomain=Discrete-time  SampleTime=-1  IntegratorMethod=Forward Euler  FilterMethod=Forward Euler  Form=Parallel  UseFilter=on  ControllerParametersSource=internal  P=1  I=1  D=0  N=100  InitialConditionSource=internal  InitialConditionForIntegrator=0  InitialConditionForFilter=0  ExternalReset=none  LimitOutput=off  UpperSaturationLimit=inf  LowerSaturationLimit=-inf  LinearizeAsGain=off  AntiWindupMode=none  Kb=1  TrackingMode=off  Kt=1  PParamMin=[]  PParamMax=[]  IParamMin=[]  IParamMax=[]  DParamMin=[]  DParamMax=[]  NParamMin=[]  NParamMax=[]  KbParamMin=[]  KbParamMax=[]  KtParamMin=[]  KtParamMax=[]  POutMin=[]  POutMax=[]  IOutMin=[]  IOutMax=[]  DOutMin=[]  DOutMax=[]  NOutMin=[]  NOutMax=[]  KbOutMin=[]  KbOutMax=[]  KtOutMin=[]  KtOutMax=[]  IntegratorOutMin=[]  IntegratorOutMax=[]  FilterOutMin=[]  FilterOutMax=[]  SumOutMin=[]  SumOutMax=[]  SumI1OutMin=[]  SumI1OutMax=[]  SumI2OutMin=[]  SumI2OutMax=[]  SumI3OutMin=[]  SumI3OutMax=[]  SumDOutMin=[]  SumDOutMax=[]  SaturationOutMin=[]  SaturationOutMax=[]  IntegratorContinuousStateAttributes=''  IntegratorStateMustResolveToSignalObject=off  IntegratorRTWStateStorageClass=Auto  FilterContinuousStateAttributes=''  FilterStateMustResolveToSignalObject=off  FilterRTWStateStorageClass=Auto  DifferentiatorICPrevScaledInput=0  DifferentiatorOutMin=[]  DifferentiatorOutMax=[]  FilterDiffOutCoefMin=[]  FilterDiffOutCoefMax=[]  SumDenOutMin=[]  SumDenOutMax=[]  SumNumOutMin=[]  SumNumOutMax=[]  ReciprocalOutMin=[]  ReciprocalOutMax=[]  DivideOutMin=[]  DivideOutMax=[]  TunerSelectOption=Transfer Function Based (PID Tuner App)
  cfblk6 : Subsystem  TreatAsAtomicUnit=on
  cfblk7 : Delay  DelayLengthSource=Input port
      settings: InputPortMap=u0,p1
  cfblk8 : simulink/Continuous/PID Controller  Controller=PID  TimeDomain=Discrete-time  SampleTime=-1  IntegratorMethod=Forward Euler  FilterMethod=Forward Euler  Form=Parallel  UseFilter=on  ControllerParametersSource=internal  P=1  I=1  D=0  N=100  InitialConditionSource=internal  InitialConditionForIntegrator=0  InitialConditionForFilter=0  ExternalReset=none  LimitOutput=off  UpperSaturationLimit=inf  LowerSaturationLimit=-inf  LinearizeAsGain=off  AntiWindupMode=none  Kb=1  TrackingMode=off  Kt=1  PParamMin=[]  PParamMax=[]  IParamMin=[]  IParamMax=[]  DParamMin=[]  DParamMax=[]  NParamMin=[]  NParamMax=[]  KbParamMin=[]  KbParamMax=[]  KtParamMin=[]  KtParamMax=[]  POutMin=[]  POutMax=[]  IOutMin=[]  IOutMax=[]  DOutMin=[]  DOutMax=[]  NOutMin=[]  NOutMax=[]  KbOutMin=[]  KbOutMax=[]  KtOutMin=[]  KtOutMax=[]  IntegratorOutMin=[]  IntegratorOutMax=[]  FilterOutMin=[]  FilterOutMax=[]  SumOutMin=[]  SumOutMax=[]  SumI1OutMin=[]  SumI1OutMax=[]  SumI2OutMin=[]  SumI2OutMax=[]  SumI3OutMin=[]  SumI3OutMax=[]  SumDOutMin=[]  SumDOutMax=[]  SaturationOutMin=[]  SaturationOutMax=[]  IntegratorContinuousStateAttributes=''  IntegratorStateMustResolveToSignalObject=off  IntegratorRTWStateStorageClass=Auto  FilterContinuousStateAttributes=''  FilterStateMustResolveToSignalObject=off  FilterRTWStateStorageClass=Auto  DifferentiatorICPrevScaledInput=0  DifferentiatorOutMin=[]  DifferentiatorOutMax=[]  FilterDiffOutCoefMin=[]  FilterDiffOutCoefMax=[]  SumDenOutMin=[]  SumDenOutMax=[]  SumNumOutMin=[]  SumNumOutMax=[]  ReciprocalOutMin=[]  ReciprocalOutMax=[]  DivideOutMin=[]  DivideOutMax=[]  TunerSelectOption=Transfer Function Based (PID Tuner App)
  cfblk9 : Delay  ShowEnablePort=on
      settings: InputPortMap=u0,e6
  cyemi_{1211..1213,1224..1226,1237..1250} (20 alike) : DataTypeConversion  OutDataTypeStr=double
  emi_1303 : Subsystem  TreatAsAtomicUnit=on
  emi_1305 : If  IfExpression=0 <= u1
  emi_1306 : DataTypeConversion  OutDataTypeStr=double
  emi_138 : Subsystem  TreatAsAtomicUnit=on
  emi_140 : If  IfExpression=0 <= u1
  emi_141 : DataTypeConversion  OutDataTypeStr=double
  emi_382 : Subsystem  TreatAsAtomicUnit=on
  emi_384 : If  IfExpression=0 <= u1
  emi_385 : DataTypeConversion  OutDataTypeStr=double
  cfblk2 : Outport
  wires:
  cfblk5/1 -> cyemi_1212/1, cyemi_1246/1
  cfblk12/1(cfblk2) -> cyemi_1211/1, cyemi_1242/1
  cfblk7/1 -> cyemi_1243/1, cyemi_1248/1, cyemi_1250/1, emi_385/1
  cfblk13/2(cfblk14) -> cfblk2/1
  cfblk11/1 -> cfblk12/Action
  cfblk11/2 -> cfblk13/Action
  cyemi_1211/1 -> cfblk10/1
  cyemi_1212/1 -> cfblk11/1
  cyemi_1213/1 -> cfblk12/1(cfblk1)
  cfblk9/1 -> cyemi_1213/1
  cyemi_1224/1 -> cfblk13/1(cfblk1)
  cyemi_1225/1 -> cfblk13/2(cfblk12)
  cfblk8/1 -> cyemi_1225/1
  cyemi_1226/1 -> cfblk13/3(cfblk13)
  cfblk14/1 -> cyemi_1226/1
  cyemi_1237/1 -> cfblk14/1
  cfblk3/1 -> cyemi_1237/1
  cyemi_1238/1 -> cfblk15/1
  cfblk13/3(cfblk15) -> cyemi_1238/1
  cfblk10/1 -> cyemi_1239/1
  cyemi_1241/1 -> cfblk3/1
  cfblk13/1(cfblk2) -> cyemi_1241/1
  cyemi_1242/1 -> cfblk4/1
  cyemi_1243/1 -> cfblk4/2
  cyemi_1244/1 -> cfblk5/1
  cfblk1/1 -> cyemi_1244/1
  cfblk4/1 -> cyemi_1245/1
  cyemi_1246/1 -> cfblk7/1
  cyemi_1247/1 -> cfblk7/2
  cfblk15/1 -> cyemi_1247/1, emi_1306/1
  cyemi_1248/1 -> cfblk8/1
  cyemi_1249/1 -> cfblk9/1
  cyemi_1250/1 -> cfblk9/2
  cyemi_1239/1 -> cfblk16/1(emi_136)
  cfblk16/1(emi_137) -> cyemi_1224/1
  emi_140/1 -> cfblk16/Action
  emi_140/2 -> emi_138/Action
  emi_141/1 -> emi_140/1
  cyemi_1245/1 -> cfblk6/1(emi_380)
  cfblk6/1(emi_381) -> cyemi_1240/1
  emi_384/1 -> cfblk6/Action
  emi_384/2 -> emi_382/Action
  emi_385/1 -> emi_384/1
  cyemi_1240/1 -> cfblk17/1(emi_1301)
  cfblk17/1(emi_1302) -> emi_141/1, cyemi_1249/1
  emi_1305/1 -> cfblk17/Action
  emi_1305/2 -> emi_1303/Action
  emi_1306/1 -> emi_1305/1

== system sampleModel7293_pp_1_1/cfblk204 ==
  cfblk1 : Inport
  cfblk11 : Inport  Port=2
  Action Port : ActionPort  ActionType=then
  cfblk10 : simulink/Discrete/Tapped Delay  vinit=0.0  samptime=-1  NumDelays=1  DelayOrder=Oldest  includeCurrent=off
  cfblk3 : Subsystem  TreatAsAtomicUnit=on
  cfblk4 : Subsystem  TreatAsAtomicUnit=on
  cfblk5 : DiscreteZeroPole  Poles=[0 0.5]  Gain=1  SampleTime=-1
  cfblk6 : DiscreteZeroPole  Poles=[0 0.5]  Gain=1  SampleTime=-1
  cfblk7 : simulink/Discrete/Difference  ICPrevInput=0.0  OutMin=[]  OutMax=[]  OutDataTypeStr=double  OutputDataTypeScalingMode=double  OutDataType=fixdt(1, 16)  OutScaling=2^-10  DoSatur=off
  cfblk8 : simulink/Discrete/Transfer Fcn Real Zero  ZeroZ=0.75  ICPrevInput=0.0  DoSatur=off
      settings: SourceProductName=Simulink  SourceProductBaseCode=SL
  cfblk9 : DiscreteFilter
  cyemi_{1253..1260} (8 alike) : DataTypeConversion  OutDataTypeStr=double
  emi_2042 : Subsystem  TreatAsAtomicUnit=on
  emi_2044 : If  IfExpression=Inf <= u1
  emi_2045 : DataTypeConversion  OutDataTypeStr=double
  emi_424 : Subsystem  TreatAsAtomicUnit=on
  emi_426 : If  IfExpression=Inf <= u1
  emi_427 : DataTypeConversion  OutDataTypeStr=double
  cfblk2 : Outport
  cfblk12 : Outport  Port=2
  cfblk13 : Outport  Port=3
  wires:
  cfblk8/1 -> cfblk2/1
  cfblk1/1 -> cfblk12/1
  cfblk6/1 -> cyemi_1254/1, cyemi_1258/1
  cfblk9/1 -> cfblk13/1
  cyemi_1253/1 -> cfblk10/1
  cfblk10/1 -> cyemi_1255/1, emi_427/1, emi_2045/1
  cyemi_1256/1 -> cfblk5/1
  cfblk7/1 -> cyemi_1256/1
  cyemi_1257/1 -> cfblk6/1
  cfblk11/1 -> cyemi_1257/1
  cyemi_1258/1 -> cfblk7/1
  cyemi_1259/1 -> cfblk8/1
  cyemi_1260/1 -> cfblk9/1
  cfblk5/1 -> cyemi_1260/1
  cyemi_1255/1 -> cfblk4/1(emi_422)
  cfblk4/1(emi_423) -> cyemi_1259/1
  emi_426/1 -> cfblk4/Action
  emi_426/2 -> emi_424/Action
  emi_427/1 -> emi_426/1
  cyemi_1254/1 -> cfblk3/1(emi_2040)
  cfblk3/1(emi_2041) -> cyemi_1253/1
  emi_2044/1 -> cfblk3/Action
  emi_2044/2 -> emi_2042/Action
  emi_2045/1 -> emi_2044/1

== system sampleModel7293_pp_1_1/cfblk205 ==
  cfblk1 : Inport
  cfblk9 : Inport  Port=2
  cfblk10 : Inport  Port=3
  Action Port : ActionPort  ActionType=else
  cfblk13 : Delay
  cfblk3 : DiscreteFir
  cfblk4 : simulink/Discrete/Transfer Fcn Lead or Lag  PoleZ=0.95  ZeroZ=0.75  ICPrevOutput=0.0  ICPrevInput=0.0  DoSatur=off
      settings: SourceProductName=Simulink  SourceProductBaseCode=SL
  cfblk5 : Subsystem  TreatAsAtomicUnit=on
  cfblk6 : DiscreteFilter
  cfblk7 : Subsystem  TreatAsAtomicUnit=on
  cfblk8 : DiscreteFilter
  cyemi_{1264..1271} (8 alike) : DataTypeConversion  OutDataTypeStr=double
  emi_1045 : Subsystem  TreatAsAtomicUnit=on
  emi_1047 : If  IfExpression=0 <= u1
  emi_1048 : DataTypeConversion  OutDataTypeStr=double
  emi_2093 : Subsystem  TreatAsAtomicUnit=on
  emi_2095 : If  IfExpression=0 <= u1
  emi_2096 : DataTypeConversion  OutDataTypeStr=double
  cfblk2 : Outport
  cfblk11 : Outport  Port=2
  cfblk12 : Outport  Port=3
  wires:
  cfblk9/1 -> cfblk12/1
  cfblk8/1 -> cfblk11/1, emi_2096/1
  cyemi_1264/1 -> cfblk13/1
  cfblk3/1 -> cyemi_1264/1
  cyemi_1265/1 -> cfblk3/1
  cyemi_1266/1 -> cfblk4/1
  cfblk1/1 -> cyemi_1266/1
  cyemi_1268/1 -> cfblk6/1
  cfblk10/1 -> cyemi_1268/1
  cfblk4/1 -> cyemi_1269/1
  cfblk13/1 -> cyemi_1270/1
  cyemi_1271/1 -> cfblk8/1
  cfblk6/1 -> cyemi_1271/1, emi_1048/1
  cyemi_1267/1 -> cfblk5/1(emi_1043)
  cfblk5/1(emi_1044) -> cfblk2/1
  emi_1047/1 -> cfblk5/Action
  emi_1047/2 -> emi_1045/Action
  emi_1048/1 -> emi_1047/1
  cyemi_1269/1 -> cfblk7/1(emi_2090)
  cyemi_1270/1 -> cfblk7/2(emi_2091)
  cfblk7/1(emi_2092) -> cyemi_1267/1, cyemi_1265/1
  emi_2095/1 -> cfblk7/Action
  emi_2095/2 -> emi_2093/Action
  emi_2096/1 -> emi_2095/1

== system sampleModel7293_pp_1_1/cfblk206 ==
  cfblk1 : Inport
  cfblk11 : Inport  Port=2
  cfblk12 : Inport  Port=3
  Action Port : ActionPort  ActionType=then
  cfblk10 : If  SampleTime=1
  cfblk16 : Subsystem  TreatAsAtomicUnit=on
  cfblk17 : Subsystem  TreatAsAtomicUnit=on
  cfblk18 : Delay
  cfblk19 : Subsystem  TreatAsAtomicUnit=on
  cfblk20 : Delay
  cfblk3 : simulink/Discrete/Difference  ICPrevInput=0.0  OutMin=[]  OutMax=[]  OutDataTypeStr=double  OutputDataTypeScalingMode=double  OutDataType=fixdt(1, 16)  OutScaling=2^-10  DoSatur=off
  cfblk4 : DiscreteIntegrator  SampleTime=-1  OutDataTypeStr=double  ICPrevOutput=DiscIntNeverNeededParam  ICPrevScaledInput=DiscIntNeverNeededParam
  cfblk5 : Delay
  cfblk6 : DiscreteStateSpace  SampleTime=-1
  cfblk7 : simulink/Discrete/Transfer Fcn First Order  PoleZ=0.95  ICPrevOutput=0.0  DoSatur=off
      settings: SourceProductName=Simulink
  cfblk8 : DiscreteTransferFcn
  cfblk9 : DiscreteTransferFcn
  cyemi_{1275..1277,1288..1289,1295..1304} (15 alike) : DataTypeConversion  OutDataTypeStr=double
  emi_2035 : Subsystem  TreatAsAtomicUnit=on
  emi_2037 : If  IfExpression=Inf <= u1
  emi_2038 : DataTypeConversion  OutDataTypeStr=double
  cfblk2 : Outport
  cfblk13 : Outport  Port=2
  cfblk14 : Outport  Port=3
  cfblk15 : Outport  Port=4
  wires:
  cfblk12/1 -> cfblk14/1
  cfblk6/1 -> cyemi_1303/1, cyemi_1304/1
  cfblk5/1 -> cfblk15/1
  cfblk16/2(cfblk13) -> cfblk13/1
  cfblk16/3(cfblk14) -> cfblk2/1
  cfblk17/1(cfblk2) -> cyemi_1295/1, cyemi_1301/1
  cfblk10/1 -> cfblk16/Action
  cfblk10/2 -> cfblk17/Action
  cyemi_1275/1 -> cfblk10/1
  cfblk18/1 -> cyemi_1275/1, emi_2038/1
  cyemi_1276/1 -> cfblk16/1(cfblk1)
  cyemi_1277/1 -> cfblk16/2(cfblk12)
  cfblk11/1 -> cyemi_1277/1
  cyemi_1288/1 -> cfblk17/1(cfblk1)
  cfblk1/1 -> cyemi_1288/1
  cyemi_1289/1 -> cfblk17/2(cfblk7)
  cfblk20/1 -> cyemi_1289/1
  cyemi_1295/1 -> cfblk18/1
  cfblk8/1 -> cyemi_1296/1
  cyemi_1297/1 -> cfblk20/1
  cfblk7/1 -> cyemi_1297/1
  cyemi_1298/1 -> cfblk3/1
  cfblk16/1(cfblk2) -> cyemi_1298/1
  cyemi_1299/1 -> cfblk4/1
  cfblk3/1 -> cyemi_1299/1
  cyemi_1300/1 -> cfblk5/1
  cfblk4/1 -> cyemi_1300/1
  cyemi_1301/1 -> cfblk6/1
  cyemi_1302/1 -> cfblk7/1
  cfblk9/1 -> cyemi_1302/1
  cyemi_1303/1 -> cfblk8/1
  cyemi_1304/1 -> cfblk9/1
  cyemi_1296/1 -> cfblk19/1(emi_2033)
  cfblk19/1(emi_2034) -> cyemi_1276/1
  emi_2037/1 -> cfblk19/Action
  emi_2037/2 -> emi_2035/Action
  emi_2038/1 -> emi_2037/1

== system sampleModel7293_pp_1_1/cfblk207 ==
  cfblk1 : Inport
  cfblk7 : Inport  Port=2
  Action Port : ActionPort  ActionType=else
  cfblk3 : simulink/Discrete/Transfer Fcn Real Zero  ZeroZ=0.75  ICPrevInput=0.0  DoSatur=off
      settings: SourceProductName=Simulink  SourceProductBaseCode=SL
  cfblk4 : simulink/Discrete/Transfer Fcn Lead or Lag  PoleZ=0.95  ZeroZ=0.75  ICPrevOutput=0.0  ICPrevInput=0.0  DoSatur=off
      settings: SourceProductName=Simulink  SourceProductBaseCode=SL
  cfblk5 : DiscreteFilter
  cfblk6 : UnitDelay  SampleTime=-1
  cyemi_{1307..1310} (4 alike) : DataTypeConversion  OutDataTypeStr=double
  cfblk2 : Outport
  wires:
  cfblk4/1 -> cfblk2/1
  cyemi_1307/1 -> cfblk3/1
  cfblk1/1 -> cyemi_1307/1
  cyemi_1308/1 -> cfblk4/1
  cfblk5/1 -> cyemi_1308/1
  cyemi_1309/1 -> cfblk5/1
  cfblk7/1 -> cyemi_1309/1
  cyemi_1310/1 -> cfblk6/1
  cfblk3/1 -> cyemi_1310/1

== system sampleModel7293_pp_1_1/cfblk208 ==
  cfblk1 : Inport
  cfblk12 : Inport  Port=2
  Action Port : ActionPort  ActionType=then
  cfblk10 : UnitDelay  SampleTime=-1
  cfblk11 : simulink/Discrete/Transfer Fcn Lead or Lag  PoleZ=0.95  ZeroZ=0.75  ICPrevOutput=0.0  ICPrevInput=0.0  DoSatur=off
      settings: SourceProductName=Simulink  SourceProductBaseCode=SL
  cfblk14 : Delay
  cfblk15 : Subsystem  TreatAsAtomicUnit=on
  cfblk16 : Delay
  cfblk3 : simulink/Continuous/PID Controller (2DOF)  Controller=PID  TimeDomain=Discrete-time  SampleTime=-1  IntegratorMethod=Forward Euler  FilterMethod=Forward Euler  Form=Parallel  UseFilter=on  ControllerParametersSource=internal  P=1  I=1  D=0  N=100  b=1  c=1  InitialConditionSource=internal  InitialConditionForIntegrator=0  InitialConditionForFilter=0  ExternalReset=none  LimitOutput=off  UpperSaturationLimit=inf  LowerSaturationLimit=-inf  LinearizeAsGain=off  AntiWindupMode=none  Kb=1  TrackingMode=off  Kt=1  PParamMin=[]  PParamMax=[]  IParamMin=[]  IParamMax=[]  DParamMin=[]  DParamMax=[]  NParamMin=[]  NParamMax=[]  bParamMin=[]  bParamMax=[]  cParamMin=[]  cParamMax=[]  KbParamMin=[]  KbParamMax=[]  KtParamMin=[]  KtParamMax=[]  POutMin=[]  POutMax=[]  IOutMin=[]  IOutMax=[]  DOutMin=[]  DOutMax=[]  NOutMin=[]  NOutMax=[]  bOutMin=[]  bOutMax=[]  cOutMin=[]  cOutMax=[]  KbOutMin=[]  KbOutMax=[]  KtOutMin=[]  KtOutMax=[]  IntegratorOutMin=[]  IntegratorOutMax=[]  FilterOutMin=[]  FilterOutMax=[]  SumOutMin=[]  SumOutMax=[]  Sum1OutMin=[]  Sum1OutMax=[]  Sum2OutMin=[]  Sum2OutMax=[]  Sum3OutMin=[]  Sum3OutMax=[]  SumI1OutMin=[]  SumI1OutMax=[]  SumI2OutMin=[]  SumI2OutMax=[]  SumI3OutMin=[]  SumI3OutMax=[]  SumDOutMin=[]  SumDOutMax=[]  SaturationOutMin=[]  SaturationOutMax=[]  IntegratorContinuousStateAttributes=''  IntegratorStateMustResolveToSignalObject=off  IntegratorRTWStateStorageClass=Auto  FilterContinuousStateAttributes=''  FilterStateMustResolveToSignalObject=off  FilterRTWStateStorageClass=Auto  DifferentiatorICPrevScaledInput=0  DifferentiatorOutMin=[]  DifferentiatorOutMax=[]  FilterDiffOutCoefMin=[]  FilterDiffOutCoefMax=[]  SumDenOutMin=[]  SumDenOutMax=[]  SumNumOutMin=[]  SumNumOutMax=[]  ReciprocalOutMin=[]  ReciprocalOutMax=[]  DivideOutMin=[]  DivideOutMax=[]  TunerSelectOption=Transfer Function Based (PID Tuner App)
  cfblk4 : UnitDelay  SampleTime=-1
  cfblk5 : DiscreteIntegrator  SampleTime=-1  OutDataTypeStr=double  ICPrevOutput=DiscIntNeverNeededParam  ICPrevScaledInput=DiscIntNeverNeededParam
  cfblk6 : Subsystem  TreatAsAtomicUnit=on
  cfblk7 : Subsystem  TreatAsAtomicUnit=on
  cfblk8 : Delay
  cfblk9 : Subsystem  TreatAsAtomicUnit=on
  cyemi_{1313..1326} (14 alike) : DataTypeConversion  OutDataTypeStr=double
  emi_1052 : Subsystem  TreatAsAtomicUnit=on
  emi_{629,1054,1568,1938} (4 alike) : If  IfExpression=Inf <= u1
  emi_{630,1055,1569,1939} (4 alike) : DataTypeConversion  OutDataTypeStr=double
  emi_1566 : Subsystem  TreatAsAtomicUnit=on
  emi_1936 : Subsystem  TreatAsAtomicUnit=on
  emi_627 : Subsystem  TreatAsAtomicUnit=on
  cfblk2 : Outport
  cfblk13 : Outport  Port=2
  wires:
  cfblk1/1 -> cfblk2/1
  cfblk3/1 -> cfblk13/1, cyemi_1320/1
  cyemi_1313/1 -> cfblk10/1
  cyemi_1314/1 -> cfblk11/1
  cyemi_1315/1 -> cfblk14/1
  cfblk5/1 -> cyemi_1315/1, emi_1939/1
  cyemi_1317/1 -> cfblk16/1
  cfblk11/1 -> cyemi_1317/1
  cyemi_1318/1 -> cfblk3/1
  cfblk14/1 -> cyemi_1318/1, emi_630/1, emi_1055/1
  cyemi_1319/1 -> cfblk3/2
  cyemi_1320/1 -> cfblk4/1
  cyemi_1321/1 -> cfblk5/1
  cfblk16/1 -> cyemi_1322/1
  cfblk4/1 -> cyemi_1323/1
  cyemi_1324/1 -> cfblk8/1
  cfblk12/1 -> cyemi_1324/1
  cfblk8/1 -> cyemi_1325/1, emi_1569/1
  cfblk10/1 -> cyemi_1326/1
  cyemi_1325/1 -> cfblk9/1(emi_624)
  cyemi_1326/1 -> cfblk9/2(emi_625)
  cfblk9/1(emi_626) -> cyemi_1321/1, cyemi_1316/1
  emi_629/1 -> cfblk9/Action
  emi_629/2 -> emi_627/Action
  emi_630/1 -> emi_629/1
  cyemi_1322/1 -> cfblk6/1(emi_1050)
  cfblk6/1(emi_1051) -> cyemi_1314/1
  emi_1054/1 -> cfblk6/Action
  emi_1054/2 -> emi_1052/Action
  emi_1055/1 -> emi_1054/1
  cyemi_1323/1 -> cfblk7/1(emi_1564)
  cfblk7/1(emi_1565) -> cyemi_1313/1
  emi_1568/1 -> cfblk7/Action
  emi_1568/2 -> emi_1566/Action
  emi_1569/1 -> emi_1568/1
  cyemi_1316/1 -> cfblk15/1(emi_1934)
  cfblk15/1(emi_1935) -> cyemi_1319/1
  emi_1938/1 -> cfblk15/Action
  emi_1938/2 -> emi_1936/Action
  emi_1939/1 -> emi_1938/1
